simulink model "kalman_filter"  (R2020a)
settings: Solver=FixedStepDiscrete  StartTime=0.0  StopTime=10.0  FixedStep=dt  RelTol=1e-3  SampleTimeConstraint=STIndependent
model workspace (MAT data in the model file):
  P0 = Simulink.Parameter
  P0.Value = [1e-06  0  0; 0  1e-06  0; 0  0  1e-06]
  P0.DataType = 'auto'
  P0.Dimensions = [3 3]
  Q = Simulink.Parameter
  Q.Value = [3.49065850399e-09  0  0; 0  3.49065850399e-09  0; 0  0  3.49065850399e-09]
  Q.Description = 'Q = dt^4/4*acceleration covariance'
  Q.DataType = 'auto'
  Q.Dimensions = [3 3]
  R = Simulink.Parameter
  R.Value = [0.0174532925199  0  0; 0  0.0174532925199  0; 0  0  0.0174532925199]
  R.Description = 'sensor covariance'
  R.DataType = 'auto'
  R.Dimensions = [3 3]
  dt = Simulink.Parameter
  dt.Value = 0.02
  dt.DataType = 'double'
  dt.Dimensions = [1 1]
  nu = Simulink.Parameter
  nu.Value = [3 1]
  nu.DataType = 'auto'
  nu.Dimensions = [1 2]
  nz = Simulink.Parameter
  nz.Value = [3 1]
  nz.DataType = 'auto'
  nz.Dimensions = [1 2]
  x0 = Simulink.Parameter
  x0.Value = [0; 0; 0]
  x0.DataType = 'auto'
  x0.Dimensions = [3 1]
values from neighbouring files (symbols this model uses):
  dt = 1/100    (= 0.01)    [load_tune.m]
  P0 = deg2rad(1)*eye(3,3)    [load_tune.m]
  Q = diag([a*pqr_dot_covar(1)*a /4, a*pqr_dot_covar(2)*a/4, a*pqr_dot_covar(3)*a/4])    [load_tune.m]
  R = diag([0.0155^2, 0.0124^2, 0.0147^2])    [load_tune.m]
  x0 = [0;0;0]    [load_tune.m]
settings Model: ParameterArgumentNames=P0,Q,R,dt,x0  OrderedModelArguments=off  Creator=Test  LastModifiedBy=Jason
settings DataIOCC: ReturnWorkspaceOutputs=off
settings DebuggingCC: AllowSymbolicDim=off  ArithmeticOperatorsInVariantConditions=warning
settings SFSimCC: SimUseLocalCustomCode=off  CustomCodeUndefinedFunction=UseInterfaceOnly
settings RTWCC: RTWUseLocalCustomCode=off

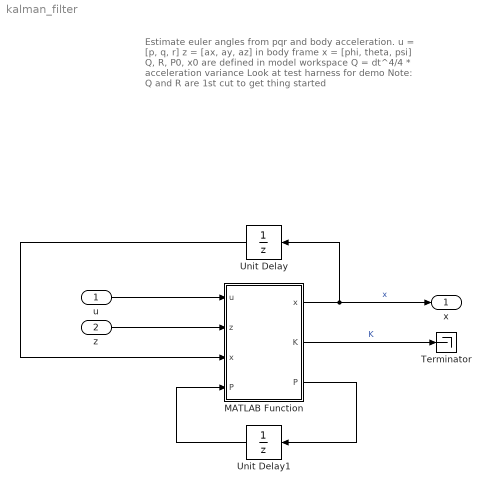
== system kalman_filter ==
  note: Estimate euler angles from pqr and body acceleration.
      |
      | u = [p, q, r]
      | z = [ax, ay, az] in body frame
      | x = [phi, theta, psi]
      |
      | Q, R, P0, x0 are defined in model workspace
      |
      | Q = dt^4/4 * acceleration variance
      |
      | Look at test harness for demo
      |
      | Note: Q and R are 1st cut to get thing started
  u : Inport  PortDimensions=nz
  z : Inport  Port=2  PortDimensions=nz
  MATLAB Function : MATLAB Function  TreatAsAtomicUnit=on  mask{Q=Q, R=R, dt=dt}
      mask prompts: dt "Sample Time"
  Terminator : Terminator
  Unit Delay : UnitDelay  InitialCondition=x0  SampleTime=-1  HasFrameUpgradeWarning=on
  Unit Delay1 : UnitDelay  InitialCondition=P0  SampleTime=-1  HasFrameUpgradeWarning=on
  x : Outport  VectorParamsAs1DForOutWhenUnconnected=off
  wires:
  MATLAB Function/1(x) -> Unit Delay/1, x/1  "x"
  Unit Delay/1 -> MATLAB Function/3("x ")
  z/1 -> MATLAB Function/2(z)
  MATLAB Function/3(P) -> Unit Delay1/1
  Unit Delay1/1 -> MATLAB Function/4("P ")
  u/1 -> MATLAB Function/1(u)
  MATLAB Function/2(K) -> Terminator/1  "K"

== matlab function kalman_filter/MATLAB Function ==
  data: u input; z input; x input; x output; K output; P output; P input; Q parameter; R parameter; dt parameter
function [x, K, P] = ekf(u, z, x, P, Q, R, dt)

[x, P] = predict(u, x, P, Q, dt);
[x, P, K] = update(z, x, P, R);

end

function [x, P] = predict(u, x, P, Q, dt)
% [x, P] = predict(u, x, P, Q, dt)
%
% predict states and covariance matrix using model

% nonlinear equation
x = eye(3,3)*x + dcm_b2e(x)*dt*u;

F = Fj();
P = F*P*F'+Q;

end

function [x, P, K] = update(z, x, P, R)
% [x, P] = update(z, x, P, R)
%
% update states and covariance matrix using measurement

g = 9.81;
dcm = dcm_i2b(x);
z_est = dcm * [0, 0, g]';
y = z - z_est;

H = Hj(x);
S = H*P*H'+R;
K = P*H'*inv(S);

nr = size(K,1);
nc = size(H,1);
x = x + K*y;
P = (eye(nr,nc)-K*H)*P;

end

function mat = Fj()
% Jacobian Matrix: F
%
% x' = Fx + Bu

mat = eye(3,3);

end

function mat = Bj(x, dt)
% Jacobian Matrix: B
%
% x' = Fx + Bu

dcm = dcm_b2e(x);
mat = dt*dcm;

end

function mat = Hj(x)
% Jacobian Matrix: H
%
% z = Hx

phi = x(1);
theta = x(2);
psi = x(3);

g = 9.81;
mat = zeros(3,3);
mat(1,2) = -cos(theta);
mat(2,1) = cos(phi)*cos(theta);
mat(2,2) = -sin(phi)*sin(theta);
mat(3,1) = -sin(phi)*cos(theta);
mat(3,2) = -cos(phi)*sin(theta);
mat = g*mat;
end
